simulink model "slosh_simulink"  (R2022b)
settings: Solver=VariableStepAuto  StartTime=0.0  StopTime=10.0  RelTol=1e-3
model workspace (MAT data in the model file):
  m = Simulink.Parameter
  m.Value = 1
  m.DataType = 'auto'
  m.Complexity = 'real'
  m.Dimensions = [1 1]
settings Model: Creator=trameshk  LastModifiedBy=trameshk

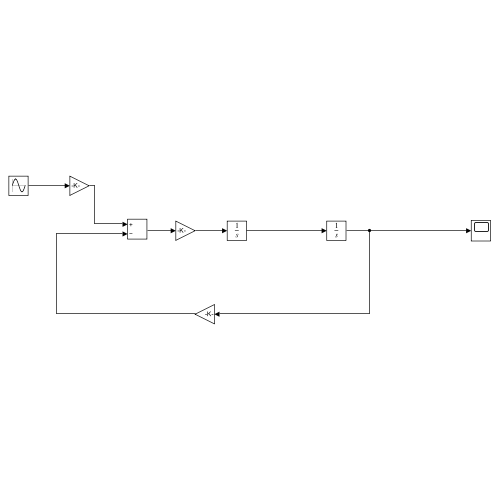
[thumbnail: Simulink's stored preview of the top-level diagram]
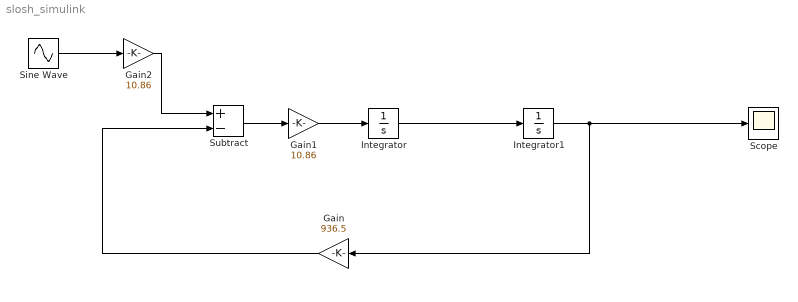
== system slosh_simulink ==
  Gain : Gain  Gain=936.5
  Gain1 : Gain  Gain=10.86
  Gain2 : Gain  Gain=10.86
  Integrator : Integrator
  Integrator1 : Integrator
  Scope : Scope
  Sine Wave : Sin  Frequency=sqrt(936.5/10.86)  SampleTime=0
  Subtract : Sum  Inputs=+-
  wires:
  Integrator/1 -> Integrator1/1
  Subtract/1 -> Gain1/1
  Sine Wave/1 -> Gain2/1
  Integrator1/1 -> Gain/1, Scope/1
  Gain1/1 -> Integrator/1
  Gain/1 -> Subtract/2
  Gain2/1 -> Subtract/1
